simulink model "pcm"  (R2018a)
settings: Solver=VariableStepAuto  StartTime=0.0  StopTime=10  RelTol=1e-3
libraries: commutil2 x2, dspquant2 x2, dsparch4 x1, dspsigops x1
settings Model: Creator=hp  LastModifiedBy=hp

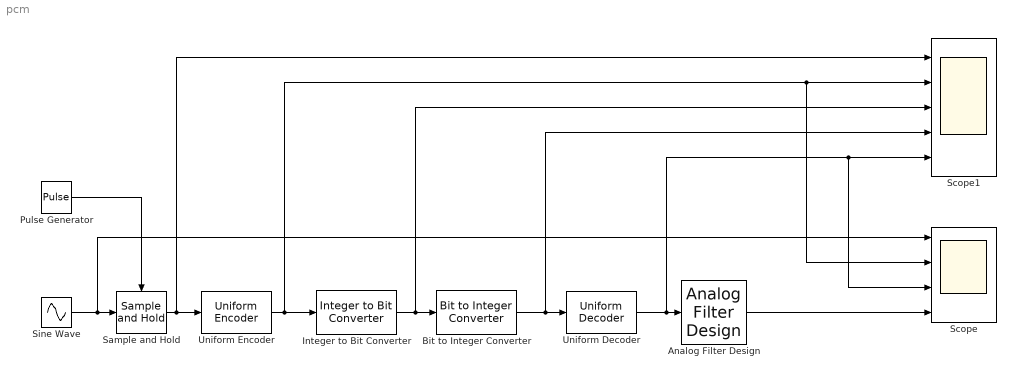
== system pcm ==
  Analog Filter Design : dsparch4/Analog Filter Design  method=Butterworth  filttype=Lowpass  N=2  Wlo=2*pi*1  Whi=80  Rp=2  Rs=40
  Bit to Integer Converter : commutil2/Bit to Integer Converter  nbits=3  bitOrder=MSB first  signedOutputValues=Unsigned  outDtype=Inherit via internal rule  outDtypeSigned=Inherit via internal rule
  Integer to Bit Converter : commutil2/Integer to Bit Converter  nbits=3  signedInputValues=Unsigned  bitOrder=MSB first  outDtype=Inherit via internal rule
  Pulse Generator : DiscretePulseGenerator  PulseType=Time based  Period=1/30  PulseWidth=50
  Sample and Hold : dspsigops/Sample and Hold  trig=Rising edge  initCond=0  latchinput=off
  Scope : Scope  NumInputPorts=4
  Scope1 : Scope  NumInputPorts=5
  Sine Wave : Sin  Frequency=2*pi*1  SampleTime=0
  Uniform Decoder : dspquant2/Uniform Decoder  peak=5  bits=3  overflowMode=Saturate  otype=Double
      settings: SourceProductName=DSP System Toolbox  SourceProductBaseCode=DS
  Uniform Encoder : dspquant2/Uniform Encoder  peak=5  bits=3  otype=Unsigned integer
      settings: SourceProductName=DSP System Toolbox
  wires:
  Sine Wave/1 -> Scope/1, Sample and Hold/1
  Pulse Generator/1 -> Sample and Hold/Trigger
  Sample and Hold/1 -> Scope1/1, Uniform Encoder/1
  Uniform Encoder/1 -> Scope/2, Scope1/2, Integer to Bit Converter/1
  Integer to Bit Converter/1 -> Scope1/3, Bit to Integer Converter/1
  Bit to Integer Converter/1 -> Scope1/4, Uniform Decoder/1
  Uniform Decoder/1 -> Scope/3, Scope1/5, Analog Filter Design/1
  Analog Filter Design/1 -> Scope/4
